simulink model "CTS_inequality_2021b"  (R2021b)
settings: Solver=FixedStepAuto  StartTime=0.0  StopTime=300  FixedStep=0.01  RelTol=1e-3
settings Model: PacingRate=0.200000  Creator=25307  LastModifiedBy=25307
settings DebuggingCC: UnconnectedInputMsg=none  UnconnectedOutputMsg=none  UnconnectedLineMsg=none
settings ModelReferenceCC: EnableRefExpFcnMdlSchedulingChecks=off
settings RTWCC: DLArmComputeVersion=20.02.1

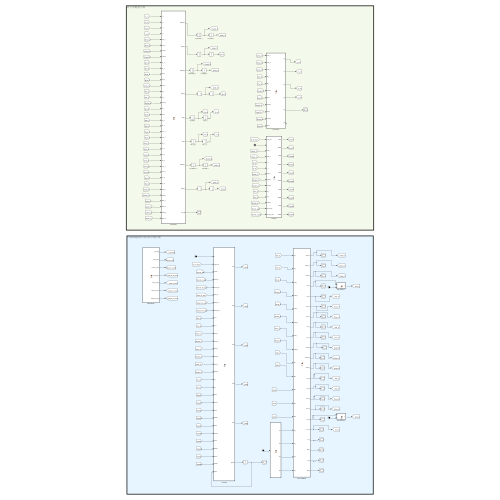
[thumbnail: Simulink's stored preview of the top-level diagram]
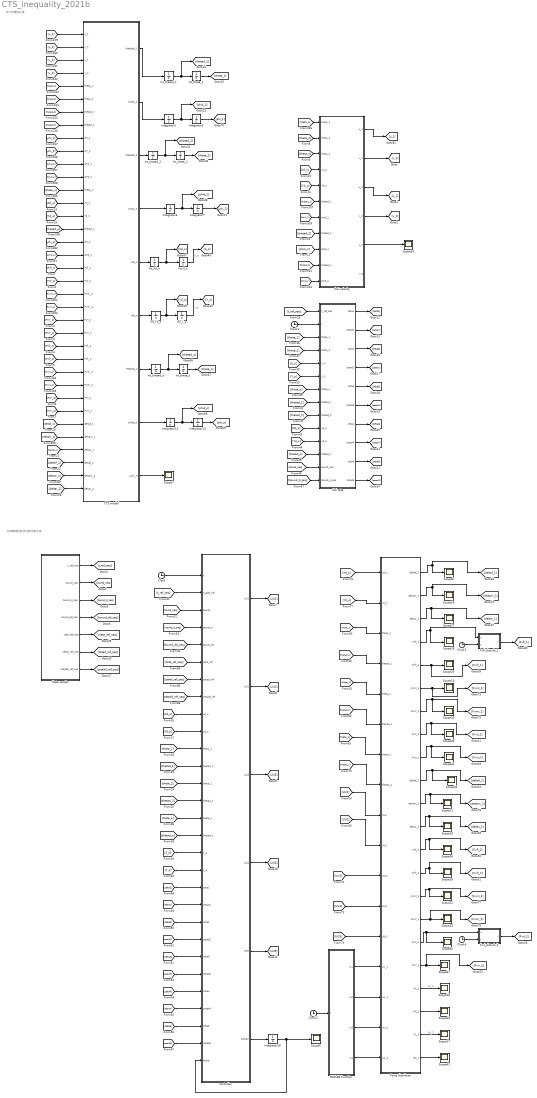
== system CTS_inequality_2021b ==
  note: 动力学模型区域
  note: 约束跟随控制及控制分配区域
  CTS model : MATLAB Function  TreatAsAtomicUnit=on
  Cal velocity : MATLAB Function  TreatAsAtomicUnit=on
  Cal zeta : MATLAB Function  TreatAsAtomicUnit=on
  Clock{,1..4} (5 alike) : Clock
  Data sender : MATLAB Function  TreatAsAtomicUnit=on
  Force distribute : MATLAB Function  TreatAsAtomicUnit=on
  Fxfl_disturb_1 : MATLAB Function  TreatAsAtomicUnit=on
  Fxrl_disturb_2 : MATLAB Function  TreatAsAtomicUnit=on
  Int_X_o : Integrator  InitialCondition=32.7448
  Int_Xd_o : Integrator  InitialCondition=1.1
  Int_Y_o : Integrator  InitialCondition=12.2889
  Int_Yd_o : Integrator  InitialCondition=0.0024
  Int_theta_1 : Integrator
  Int_theta_2 : Integrator  InitialCondition=0.005
  Int_theta_o : Integrator  InitialCondition=0.0014
  Int_thetad_1 : Integrator
  Int_thetad_2 : Integrator  InitialCondition=-0.0031
  Int_thetad_o : Integrator  InitialCondition=-0.001
  Integrator{2..3,6..7,12..13} (6 alike) : Integrator
  Integrator16 : Integrator  InitialCondition=0.5
  MATLAB Function : MATLAB Function  TreatAsAtomicUnit=on
  Scope{5..7,16..24,27..37,40..41} (25 alike) : Scope
  controller : MATLAB Function  TreatAsAtomicUnit=on
  wires:
  [theta_o] -> Cal velocity/3(theta_o)
  [thetad_1] -> CTS model/7(thetad_1)
  [theta_o] -> CTS model/13(theta_o)
  [theta_2] -> CTS model/6(theta_2)
  [phid_1] -> Cal velocity/7(phid_1)
  [Fxrl_1] -> CTS model/23(Fxrl_1)
  Integrator6/1 -> [phid_2], Integrator7/1
  [Fxfr_2] -> CTS model/26(Fxfr_2)
  [phi_o] -> CTS model/17(phi_o)
  [deltaf_2] -> CTS model/34(deltaf_2)
  [Yd_o] -> Cal velocity/5(Yd_o)
  [phi_2] -> CTS model/10(phi_2)
  [theta_1] -> Cal velocity/1(theta_1)
  [Fxrl_2] -> CTS model/29(Fxrl_2)
  [theta_2] -> Cal velocity/2(theta_2)
  [phid_1] -> CTS model/11(phid_1)
  Integrator3/1 -> [phi_1]
  [v_1] -> CTS model/3(v_1)
  CTS model/8(phidd_o) -> Integrator12/1
  [Xd_o] -> Cal velocity/4(Xd_o)
  [thetad_2] -> CTS model/8(thetad_2)
  [phid_2] -> Cal velocity/9(phid_2)
  [phid_2] -> CTS model/12(phid_2)
  [Xd_o] -> CTS model/14(Xd_o)
  Cal velocity/2(v_1) -> [v_1]
  [thetad_1] -> Cal velocity/6(thetad_1)
  [deltar_1] -> CTS model/33(deltar_1)
  Cal velocity/4(v_2) -> [v_2]
  [u_1] -> CTS model/1(u_1)
  Integrator12/1 -> [phid_o], Integrator13/1
  [Fxfl_1] -> CTS model/19(Fxfl_1)
  [Fxrr_2] -> CTS model/30(Fxrr_2)
  [deltaf_1] -> CTS model/31(deltaf_1)
  [thetad_o] -> Cal velocity/10(thetad_o)
  [Fxrr_1] -> CTS model/24(Fxrr_1)
  Cal velocity/1(u_1) -> [u_1]
  Integrator13/1 -> [phi_o]
  [phid_o] -> CTS model/18(phid_o)
  CTS model/4(phidd_2) -> Integrator6/1
  CTS model/9(rank_M) -> Scope7/1
  Integrator7/1 -> [phi_2]
  [u_2] -> CTS model/2(u_2)
  [Fxfl_2] -> CTS model/25(Fxfl_2)
  [thetad_2] -> Cal velocity/8(thetad_2)
  [v_2] -> CTS model/4(v_2)
  [Yd_o] -> CTS model/15(Yd_o)
  [phi_1] -> CTS model/9(phi_1)
  [theta_1] -> CTS model/5(theta_1)
  [thetad_o] -> CTS model/16(thetad_o)
  Integrator2/1 -> [phid_1], Integrator3/1
  [deltar_2] -> CTS model/36(deltar_2)
  CTS model/2(phidd_1) -> Integrator2/1
  [Fxfr_1] -> CTS model/20(Fxfr_1)
  [phid_o] -> Cal velocity/11(phid_o)
  Cal velocity/3(u_2) -> [u_2]
  [bound_d_seq] -> controller/4(bound_d)
  [zetadd_ref_seq] -> controller/8(zetadd_ref)
  [bound_dd_seq] -> controller/5(bound_dd)
  controller/6(alphad) -> Integrator16/1
  Data sender/5(zeta_ref_seq) -> [zeta_ref_seq]
  [zetad2] -> controller/22(zetad2)
  Data sender/7(zetadd_ref_seq) -> [zetadd_ref_seq]
  [theta_o] -> Force distribute/7(theta_o)
  Data sender/6(zetad_ref_seq) -> [zetad_ref_seq]
  [theta_1] -> Force distribute/3(theta_1)
  [zeta_ref_seq] -> controller/6(zeta_ref)
  [zetad_ref_seq] -> controller/7(zetad_ref)
  Force distribute/4(Fxfl_1) -> Scope28/1, Fxfl_disturb_1/1(u)
  Data sender/3(bound_d_seq) -> [bound_d_seq]
  [zetad4] -> controller/26(zetad4)
  [zetad3] -> controller/24(zetad3)
  controller/4(UU4) -> [UU4]
  Clock/1 -> controller/1(t)
  [zetad5] -> controller/28(zetad5)
  [bound_seq] -> controller/3(bound)
  [thetad_o] -> Force distribute/8(thetad_o)
  [zeta3] -> controller/23(zeta3)
  Integrator16/1 -> Scope5/1, controller/29(alpha)
  [zeta4] -> controller/25(zeta4)
  [UU5] -> Force distribute/13(UU5)
  controller/5(UU5) -> [UU5]
  [theta_o] -> controller/15(theta_o)
  [X_o] -> controller/17(x_o)
  [zeta1] -> controller/19(zeta1)
  controller/3(UU3) -> [UU3]
  Data sender/1(t_ref_seq) -> [t_ref_seq]
  [t_ref_seq] -> controller/2(t_glob_ref)
  Force distribute/1(deltaf_1) -> Scope6/1, [deltaf_1]
  [thetad_2] -> controller/14(thetad_2)
  [theta_1] -> controller/11(theta_1)
  [Xd_o] -> controller/9(xd_o)
  Force distribute/12(deltar_2) -> Scope33/1, [deltar_2]
  [Y_o] -> controller/18(y_o)
  [thetad_1] -> controller/12(thetad_1)
  [Yd_o] -> controller/10(yd_o)
  Data sender/2(bound_seq) -> [bound_seq]
  [thetad_1] -> Force distribute/4(thetad_1)
  controller/1(UU1) -> [UU1]
  Force distribute/5(Fxfr_1) -> [Fxfr_1], Scope29/1
  Force distribute/18(Fxrr_2) -> [Fxrr_2], Scope37/1
  [theta_2] -> controller/13(theta_2)
  [UU4] -> Force distribute/12(UU4)
  [UU3] -> Force distribute/11(UU3)
  Force distribute/9(Fxrr_1) -> Scope31/1, [Fxrr_1]
  [zeta5] -> controller/27(zeta5)
  Force distribute/10(deltaf_2) -> Scope32/1, [deltaf_2]
  [UU1] -> Force distribute/9(UU1)
  [zetad1] -> controller/20(zetad1)
  [zeta2] -> controller/21(zeta2)
  [thetad_2] -> Force distribute/6(thetad_2)
  [Yd_o] -> Force distribute/2(yd_o)
  [thetad_o] -> controller/16(thetad_o)
  Force distribute/8(Fxrl_1) -> Scope30/1, [Fxrl_1]
  Data sender/4(bound_dd_seq) -> [bound_dd_seq]
  Force distribute/14(Fxfr_2) -> Scope35/1, [Fxfr_2]
  controller/2(UU2) -> [UU2]
  Force distribute/13(Fxfl_2) -> Scope34/1, [Fxfl_2]
  [theta_2] -> Force distribute/5(theta_2)
  [Xd_o] -> Force distribute/1(xd_o)
  [UU2] -> Force distribute/10(UU2)
  Cal zeta/3(zeta2) -> [zeta2]
  Cal zeta/10(zetad5) -> [zetad5]
  [t_ref_seq] -> Cal zeta/1(t_ref_seq)
  Cal zeta/8(zetad4) -> [zetad4]
  [Xd_o] -> Cal zeta/10(xd_o)
  [theta_2] -> Cal zeta/4(theta_2)
  [theta_o] -> Cal zeta/7(theta_o)
  Cal zeta/7(zeta4) -> [zeta4]
  Cal zeta/2(zetad1) -> [zetad1]
  [Yd_o] -> Cal zeta/11(yd_o)
  [X_o] -> Cal zeta/5(x_o)
  Cal zeta/1(zeta1) -> [zeta1]
  [thetad_2] -> Cal zeta/9(thetad_2)
  [bound_d_seq] -> Cal zeta/14(bound_d_seq)
  [thetad_1] -> Cal zeta/8(thetad_1)
  Cal zeta/9(zeta5) -> [zeta5]
  [Y_o] -> Cal zeta/6(y_o)
  [bound_seq] -> Cal zeta/13(bound_seq)
  Cal zeta/5(zeta3) -> [zeta3]
  Cal zeta/4(zetad2) -> [zetad2]
  [thetad_o] -> Cal zeta/12(thetad_o)
  [theta_1] -> Cal zeta/3(theta_1)
  Clock1/1 -> Cal zeta/2(t)
  Cal zeta/6(zetad3) -> [zetad3]
  Int_theta_1/1 -> [theta_1]
  CTS model/1(thetadd_1) -> Int_thetad_1/1
  Int_thetad_1/1 -> [thetad_1], Int_theta_1/1
  Int_thetad_2/1 -> [thetad_2], Int_theta_2/1
  Int_theta_2/1 -> [theta_2]
  CTS model/3(thetadd_2) -> Int_thetad_2/1
  CTS model/5(Xdd_o) -> Int_Xd_o/1
  Int_Xd_o/1 -> Int_X_o/1, [Xd_o]
  Int_X_o/1 -> [X_o]  "X_o"
  Int_Y_o/1 -> [Y_o]  "Y_o"
  Int_Yd_o/1 -> Int_Y_o/1, [Yd_o]
  CTS model/6(Ydd_o) -> Int_Yd_o/1
  CTS model/7(thetadd_o) -> Int_thetad_o/1
  Int_thetad_o/1 -> [thetad_o], Int_theta_o/1
  Int_theta_o/1 -> [theta_o]
  MATLAB Function/1(w1) -> Force distribute/14(wx_1)
  MATLAB Function/2(w2) -> Force distribute/15(wz_1)
  MATLAB Function/3(w3) -> Force distribute/16(wx_2)
  MATLAB Function/4(w4) -> Force distribute/17(wz_2)
  Clock2/1 -> MATLAB Function/1(t)
  Clock3/1 -> Fxfl_disturb_1/2(t)
  Fxfl_disturb_1/1(y) -> [Fxfl_1]
  Clock4/1 -> Fxrl_disturb_2/2(t)
  Fxrl_disturb_2/1(y) -> [Fxrl_2]
  Force distribute/17(Fxrl_2) -> Scope36/1, Fxrl_disturb_2/1(u)
  Force distribute/19(Fx_1) -> Scope16/1  "Fx_1"
  Force distribute/21(Fx_2) -> Scope17/1  "Fx_2"
  Force distribute/2(deltam_1) -> Scope18/1, [deltam_1]
  Force distribute/7(Fxmr_1) -> Scope20/1, [Fxmr_1]
  Force distribute/6(Fxml_1) -> Scope19/1, [Fxml_1]
  Force distribute/11(deltam_2) -> Scope21/1, [deltam_2]
  Force distribute/15(Fxml_2) -> Scope22/1, [Fxml_2]
  Force distribute/16(Fxmr_2) -> [Fxmr_2], Scope23/1
  [Fxml_1] -> CTS model/21(Fxml_1)
  [Fxmr_1] -> CTS model/22(Fxmr_1)
  [Fxml_2] -> CTS model/27(Fxml_2)
  [Fxmr_2] -> CTS model/28(Fxmr_2)
  [deltam_1] -> CTS model/32(deltam_1)
  [deltam_2] -> CTS model/35(deltam_2)
  Cal velocity/5(u_o) -> Scope24/1
  Force distribute/3(deltar_1) -> Scope27/1, [deltar_1]
  Force distribute/20(MZ_1) -> Scope40/1
  Force distribute/22(MZ_2) -> Scope41/1

== matlab function CTS_inequality_2021b/Cal zeta ==
  data: t_ref_seq input; zeta1 output; t input; theta_1 input; theta_2 input; x_o input; y_o input; theta_o input; thetad_1 input; thetad_2 input; xd_o input; yd_o input; thetad_o input; bound_seq input; bound_d_seq input; zetad1 output; zeta2 output; zetad2 output; zeta3 output; zetad3 output; zeta4 output; zetad4 output; zeta5 output; zetad5 output
function [zeta1,zetad1,zeta2,zetad2,zeta3,zetad3,zeta4,zetad4,zeta5,zetad5] = fcn(t_ref_seq,t,theta_1,theta_2,x_o,y_o,theta_o,thetad_1,thetad_2,xd_o,yd_o,thetad_o,bound_seq,bound_d_seq)

x_hi_all_o = bound_seq(1,:);
x_lo_all_o = bound_seq(2,:);
y_hi_all_o = bound_seq(3,:);
y_lo_all_o = bound_seq(4,:);
theta_hi_all_o = bound_seq(5,:);
theta_lo_all_o = bound_seq(6,:);
theta_hi_all_1 = bound_seq(7,:);
theta_lo_all_1 = bound_seq(8,:);
theta_hi_all_2 = bound_seq(9,:);
theta_lo_all_2 = bound_seq(10,:);

xd_hi_all_o = bound_d_seq(1,:);
xd_lo_all_o = bound_d_seq(2,:);
yd_hi_all_o = bound_d_seq(3,:);
yd_lo_all_o = bound_d_seq(4,:);
thetad_hi_all_o = bound_d_seq(5,:);
thetad_lo_all_o = bound_d_seq(6,:);
thetad_hi_all_1 = bound_d_seq(7,:);
thetad_lo_all_1 = bound_d_seq(8,:);
thetad_hi_all_2 = bound_d_seq(9,:);
thetad_lo_all_2 = bound_d_seq(10,:);


x_hi_o = spline(t_ref_seq,x_hi_all_o,t);
x_lo_o = spline(t_ref_seq,x_lo_all_o,t);
y_hi_o = spline(t_ref_seq,y_hi_all_o,t);
y_lo_o = spline(t_ref_seq,y_lo_all_o,t);
theta_hi_o = spline(t_ref_seq,theta_hi_all_o,t);
theta_lo_o = spline(t_ref_seq,theta_lo_all_o,t);
theta_hi_1 = spline(t_ref_seq,theta_hi_all_1,t);
theta_lo_1 = spline(t_ref_seq,theta_lo_all_1,t);
theta_hi_2 = spline(t_ref_seq,theta_hi_all_2,t);
theta_lo_2 = spline(t_ref_seq,theta_lo_all_2,t);

xd_hi_o = spline(t_ref_seq,xd_hi_all_o,t);
xd_lo_o = spline(t_ref_seq,xd_lo_all_o,t);
yd_hi_o = spline(t_ref_seq,yd_hi_all_o,t);
yd_lo_o = spline(t_ref_seq,yd_lo_all_o,t);
thetad_hi_o = spline(t_ref_seq,thetad_hi_all_o,t);
thetad_lo_o = spline(t_ref_seq,thetad_lo_all_o,t);
thetad_hi_1 = spline(t_ref_seq,thetad_hi_all_1,t);
thetad_lo_1 = spline(t_ref_seq,thetad_lo_all_1,t);
thetad_hi_2 = spline(t_ref_seq,thetad_hi_all_2,t);
thetad_lo_2 = spline(t_ref_seq,thetad_lo_all_2,t);

zeta1 = log((theta_1-theta_lo_1)/(theta_hi_1-theta_1));
zeta2 = log((theta_2-theta_lo_2)/(theta_hi_2-theta_2));
zeta3 = log((x_o-x_lo_o)/(x_hi_o-x_o));
zeta4 = log((y_o-y_lo_o)/(y_hi_o-y_o));
zeta5 = log((theta_o-theta_lo_o)/(theta_hi_o-theta_o));

zetad1 = (((thetad_1-thetad_lo_1)/(theta_1-theta_hi_1)-((thetad_1-thetad_hi_1)*(theta_1-theta_lo_1))/(theta_1-theta_hi_1)^2)*(theta_1-theta_hi_1))/(theta_1-theta_lo_1);
zetad2 = (((thetad_2-thetad_lo_2)/(theta_2-theta_hi_2)-((thetad_2-thetad_hi_2)*(theta_2-theta_lo_2))/(theta_2-theta_hi_2)^2)*(theta_2-theta_hi_2))/(theta_2-theta_lo_2);
zetad3 = (((xd_o-xd_lo_o)/(x_o-x_hi_o)-((xd_o-xd_hi_o)*(x_o-x_lo_o))/(x_o-x_hi_o)^2)*(x_o-x_hi_o))/(x_o-x_lo_o);
zetad4 = (((yd_o-yd_lo_o)/(y_o-y_hi_o)-((yd_o-yd_hi_o)*(y_o-y_lo_o))/(y_o-y_hi_o)^2)*(y_o-y_hi_o))/(y_o-y_lo_o);
zetad5 = (((thetad_o-thetad_lo_o)/(theta_o-theta_hi_o)-((thetad_o-thetad_hi_o)*(theta_o-theta_lo_o))/(theta_o-theta_hi_o)^2)*(theta_o-theta_hi_o))/(theta_o-theta_lo_o);

== matlab function CTS_inequality_2021b/CTS model ==
  data: thetadd_1 output; phidd_1 output; thetadd_2 output; phidd_2 output; Xdd_o output; Ydd_o output; thetadd_o output; phidd_o output; u_1 input; u_2 input; v_1 input; v_2 input; theta_1 input; theta_2 input; thetad_1 input; thetad_2 input; phi_1 input; phi_2 input; phid_1 input; phid_2 input; theta_o input; Xd_o input; Yd_o input; thetad_o input; phi_o input; phid_o input; Fxfl_1 input; Fxfr_1 input; Fxml_1 input; Fxmr_1 input; Fxrl_1 input; Fxrr_1 input; Fxfl_2 input; Fxfr_2 input; Fxml_2 input; Fxmr_2 input; Fxrl_2 input; Fxrr_2 input; rank_M output; deltaf_1 input; deltam_1 input; deltar_1 input; deltaf_2 input; deltam_2 input; deltar_2 input
function [thetadd_1,phidd_1,thetadd_2,phidd_2,Xdd_o,Ydd_o,thetadd_o,phidd_o,rank_M] = fcn(u_1,u_2,v_1,v_2,theta_1,theta_2,thetad_1,thetad_2,phi_1,phi_2,phid_1,phid_2,theta_o,Xd_o,Yd_o,thetad_o,phi_o,phid_o,...
    Fxfl_1,Fxfr_1,Fxml_1,Fxmr_1,Fxrl_1,Fxrr_1,Fxfl_2,Fxfr_2,Fxml_2,Fxmr_2,Fxrl_2,Fxrr_2,deltaf_1,deltam_1,deltar_1,deltaf_2,deltam_2,deltar_2)



m_1 = 4455;
Iz_1 = 26802.6;
a_1 = 1.11;
b_1 = 0.12;
c_1 = 1.23;
d_1 = 0.5;
r_1 = 5;
phip_1 = 0;
Cf_1 = -87752;
Cm_1 = -82100;
Cr_1 = -88752;
ms_1 = 4155;
Ix_1 = 2283.9;
K_1 = 253750;
C_1 = 15225;
hs_1 = 0.65;
hcr_1 = 1;


m_2 = 5925;
Iz_2 = 24802.6;
a_2 = 1.11;
b_2 = 0.12;
c_2 = 1.23;
d_2 = 0.5;
r_2 = 5;
phip_2 = pi;
Cf_2 = -86752;
Cm_2 = -83222;
Cr_2 = -85752;
ms_2 = 5455;
Ix_2 = 2283.9;
K_2 = 253750;
C_2 = 15225;
hs_2 = 0.65;
hcr_2 = 1;

m_o = 5925;
Iz_o = 65992;
Ix_o = 4690;
H_o = 1.5;
Kj = 333023;
Cj = 45023;
g = 9.81;

T_1 = 1.5;
T_2 = 1.5;

hr = 0.2;


Fx_1 = Fxfl_1+Fxfr_1+Fxml_1+Fxmr_1+Fxrl_1+Fxrr_1;
Fy_1 = (Fxfl_1+Fxfr_1)*deltaf_1+(Fxml_1+Fxmr_1)*deltam_1+(Fxrl_1+Fxrr_1)*deltar_1;
Mz_1 = (Fxfl_1+Fxfr_1)*a_1*deltaf_1-(Fxfl_1-Fxfr_1)*T_1/2-(Fxml_1+Fxmr_1)*b_1*deltam_1-(Fxml_1-Fxmr_1)*T_1/2-(Fxrl_1+Fxrr_1)*c_1*deltar_1-(Fxrl_1-Fxrr_1)*T_1/2;

Q1_1 = m_1*v_1*thetad_1;
Q2_1 = -m_1*u_1*thetad_1+2*Cf_1*(v_1+thetad_1*a_1)/u_1+2*Cm_1*(v_1-thetad_1*b_1)/u_1+2*Cr_1*(v_1-thetad_1*c_1)/u_1;
Q3_1 = 2*Cf_1*(v_1+thetad_1*a_1)/u_1*a_1-2*Cm_1*(v_1-thetad_1*b_1)/u_1*b_1-2*Cr_1*(v_1-thetad_1*c_1)/u_1*c_1;
Q4_1 = -K_1*phi_1-C_1*phid_1+ms_1*g*(hs_1-hr)*phi_1+ms_1*(hs_1-hr)*u_1*thetad_1+Kj*(phi_o-phi_1)+Cj*(phid_o-phid_1);

U1_1 = -2*Cf_1*(v_1+thetad_1*a_1)/u_1*deltaf_1-2*Cm_1*(v_1-thetad_1*b_1)/u_1*deltam_1-2*Cr_1*(v_1-thetad_1*c_1)/u_1*deltar_1+Fx_1+2*(Cf_1*deltaf_1^2+Cm_1*deltam_1^2+Cr_1*deltar_1^2);
U2_1 = -2*Cf_1*deltaf_1-2*Cm_1*deltam_1-2*Cr_1*deltar_1+Fy_1;
U3_1 = -2*Cf_1*a_1*deltaf_1+2*Cm_1*b_1*deltam_1+2*Cr_1*c_1*deltar_1+Mz_1;


Fx_2 = Fxfl_2+Fxfr_2+Fxml_2+Fxmr_2+Fxrl_2+Fxrr_2;
Fy_2 = (Fxfl_2+Fxfr_2)*deltaf_2+(Fxml_2+Fxmr_2)*deltam_2+(Fxrl_2+Fxrr_2)*deltar_2;
Mz_2 = (Fxfl_2+Fxfr_2)*a_2*deltaf_2-(Fxfl_2-Fxfr_2)*T_2/2-(Fxml_2+Fxmr_2)*b_2*deltam_2-(Fxml_2-Fxmr_2)*T_2/2-(Fxrl_2+Fxrr_2)*c_2*deltar_2-(Fxrl_2-Fxrr_2)*T_2/2;

Q1_2 = m_2*v_2*thetad_2;
Q2_2 = -m_2*u_2*thetad_2+2*Cf_2*(v_2+thetad_2*a_2)/u_2+2*Cm_2*(v_2-thetad_2*b_2)/u_2+2*Cr_2*(v_2-thetad_2*c_2)/u_2;
Q3_2 = 2*Cf_2*(v_2+thetad_2*a_2)/u_2*a_2-2*Cm_2*(v_2-thetad_2*b_2)/u_2*b_2-2*Cr_2*(v_2-thetad_2*c_2)/u_2*c_2;
Q4_2 = -K_2*phi_2-C_2*phid_2+ms_2*g*(hs_2-hr)*phi_2+ms_2*(hs_2-hr)*u_2*thetad_2+Kj*(phi_o-phi_2)+Cj*(phid_o-phid_2);

U1_2 = -2*Cf_2*(v_2+thetad_2*a_2)/u_2*deltaf_2-2*Cm_2*(v_2-thetad_2*b_2)/u_2*deltam_2-2*Cr_2*(v_2-thetad_2*c_2)/u_2*deltar_2+Fx_2+2*(Cf_2*deltaf_2^2+Cm_2*deltam_2^2+Cr_2*deltar_2^2);
U2_2 = -2*Cf_2*deltaf_2-2*Cm_2*deltam_2-2*Cr_2*deltar_2+Fy_2;
U3_2 = -2*Cf_2*a_2*deltaf_2+2*Cm_2*b_2*deltam_2+2*Cr_2*c_2*deltar_2+Mz_2;

Q4_o = -Kj*(phi_o-phi_1)-Kj*(phi_o-phi_2)-Cj*(phid_o-phid_1)-Cj*(phid_o-phid_2)+m_o*g*(H_o-hr)*phi_o;


M = zeros(8,8);
M(1,1) = (m_1*d_1^2+Iz_1);
M(1,2) = +(d_1*hr*m_1-d_1*hcr_1*m_1-d_1*hr*ms_1+d_1*hs_1*ms_1);
M(1,3) = 0;
M(1,4) = 0;
M(1,5) = +(d_1*m_1*sin(theta_1));
M(1,6) = +(-d_1*m_1*cos(theta_1));
M(1,7) = +(-d_1*m_1*r_1*cos(phip_1-theta_1+theta_o));
M(1,8) = +(d_1*hcr_1*m_1*cos(theta_1-theta_o)-d_1*hr*m_1*cos(theta_1-theta_o));

M(2,1) = (d_1*hr*m_1-d_1*hcr_1*m_1-d_1*hr*ms_1+d_1*hs_1*ms_1);
M(2,2) = +(Ix_1+hcr_1^2*m_1+hr^2*m_1-hr^2*ms_1+hs_1^2*ms_1-2*hcr_1*hr*m_1+2*hcr_1*hr*ms_1-2*hcr_1*hs_1*ms_1);
M(2,3) = 0;
M(2,4) = 0;
M(2,5) = +(hr*m_1*sin(theta_1)-hcr_1*m_1*sin(theta_1)-hr*ms_1*sin(theta_1)+hs_1*ms_1*sin(theta_1));
M(2,6) = +(hcr_1*m_1*cos(theta_1)-hr*m_1*cos(theta_1)+hr*ms_1*cos(theta_1)-hs_1*ms_1*cos(theta_1));
M(2,7) = +(hcr_1*m_1*r_1*cos(phip_1-theta_1+theta_o)-hr*m_1*r_1*cos(phip_1-theta_1+theta_o)+hr*ms_1*r_1*cos(phip_1-theta_1+theta_o)-hs_1*ms_1*r_1*cos(phip_1-theta_1+theta_o));
M(2,8) = +(hr^2*ms_1*cos(theta_1-theta_o)-hr^2*m_1*cos(theta_1-theta_o)-hcr_1^2*m_1*cos(theta_1-theta_o)+2*hcr_1*hr*m_1*cos(theta_1-theta_o)-hcr_1*hr*ms_1*cos(theta_1-theta_o)+hcr_1*hs_1*ms_1*cos(theta_1-theta_o)-hr*hs_1*ms_1*cos(theta_1-theta_o));

M(3,1) = 0;
M(3,2) = 0;
M(3,3) = (m_2*d_2^2+Iz_2);
M(3,4) = +(d_2*hr*m_2-d_2*hcr_2*m_2-d_2*hr*ms_2+d_2*hs_2*ms_2);
M(3,5) = +(d_2*m_2*sin(theta_2));
M(3,6) = +(-d_2*m_2*cos(theta_2));
M(3,7) = +(-d_2*m_2*r_2*cos(phip_2-theta_2+theta_o));
M(3,8) = +(d_2*hcr_2*m_2*cos(theta_2-theta_o)-d_2*hr*m_2*cos(theta_2-theta_o));

M(4,1) = 0;
M(4,2) = 0;
M(4,3) = (d_2*hr*m_2-d_2*hcr_2*m_2-d_2*hr*ms_2+d_2*hs_2*ms_2);
M(4,4) = +(Ix_2+hcr_2^2*m_2+hr^2*m_2-hr^2*ms_2+hs_2^2*ms_2-2*hcr_2*hr*m_2+2*hcr_2*hr*ms_2-2*hcr_2*hs_2*ms_2);
M(4,5) = +(hr*m_2*sin(theta_2)-hcr_2*m_2*sin(theta_2)-hr*ms_2*sin(theta_2)+hs_2*ms_2*sin(theta_2));
M(4,6) = +(hcr_2*m_2*cos(theta_2)-hr*m_2*cos(theta_2)+hr*ms_2*cos(theta_2)-hs_2*ms_2*cos(theta_2));
M(4,7) = +(hcr_2*m_2*r_2*cos(phip_2-theta_2+theta_o)-hr*m_2*r_2*cos(phip_2-theta_2+theta_o)+hr*ms_2*r_2*cos(phip_2-theta_2+theta_o)-hs_2*ms_2*r_2*cos(phip_2-theta_2+theta_o));
M(4,8) = +(hr^2*ms_2*cos(theta_2-theta_o)-hr^2*m_2*cos(theta_2-theta_o)-hcr_2^2*m_2*cos(theta_2-theta_o)+2*hcr_2*hr*m_2*cos(theta_2-theta_o)-hcr_2*hr*ms_2*cos(theta_2-theta_o)+hcr_2*hs_2*ms_2*cos(theta_2-theta_o)-hr*hs_2*ms_2*cos(theta_2-theta_o));

M(5,1) = (d_1*m_1*sin(theta_1));
M(5,2) = +(hr*m_1*sin(theta_1)-hcr_1*m_1*sin(theta_1)-hr*ms_1*sin(theta_1)+hs_1*ms_1*sin(theta_1));
M(5,3) = +(d_2*m_2*sin(theta_2));
M(5,4) = +(hr*m_2*sin(theta_2)-hcr_2*m_2*sin(theta_2)-hr*ms_2*sin(theta_2)+hs_2*ms_2*sin(theta_2));
M(5,5) = +(m_1+m_2+m_o);
M(5,6) = 0;
M(5,7) = +(-m_1*r_1*sin(phip_1+theta_o)-m_2*r_2*sin(phip_2+theta_o));
M(5,8) = +(hcr_1*m_1*sin(theta_o)+hcr_2*m_2*sin(theta_o)-hr*m_1*sin(theta_o)-hr*m_2*sin(theta_o)-hr*m_o*sin(theta_o)+H_o*m_o*sin(theta_o));

M(6,1) = (-d_1*m_1*cos(theta_1));
M(6,2) = +(hcr_1*m_1*cos(theta_1)-hr*m_1*cos(theta_1)+hr*ms_1*cos(theta_1)-hs_1*ms_1*cos(theta_1));
M(6,3) = +(-d_2*m_2*cos(theta_2));
M(6,4) = +(hcr_2*m_2*cos(theta_2)-hr*m_2*cos(theta_2)+hr*ms_2*cos(theta_2)-hs_2*ms_2*cos(theta_2));
M(6,5) = 0;
M(6,6) = +(m_1+m_2+m_o);
M(6,7) = +(m_1*r_1*cos(phip_1+theta_o)+m_2*r_2*cos(phip_2+theta_o));
M(6,8) = +(hr*m_1*cos(theta_o)-hcr_2*m_2*cos(theta_o)-hcr_1*m_1*cos(theta_o)+hr*m_2*cos(theta_o)+hr*m_o*cos(theta_o)-H_o*m_o*cos(theta_o));

M(7,1) = (-d_1*m_1*r_1*cos(phip_1-theta_1+theta_o));
M(7,2) = +(hcr_1*m_1*r_1*cos(phip_1-theta_1+theta_o)-hr*m_1*r_1*cos(phip_1-theta_1+theta_o)+hr*ms_1*r_1*cos(phip_1-theta_1+theta_o)-hs_1*ms_1*r_1*cos(phip_1-theta_1+theta_o));
M(7,3) = +(-d_2*m_2*r_2*cos(phip_2-theta_2+theta_o));
M(7,4) = +(hcr_2*m_2*r_2*cos(phip_2-theta_2+theta_o)-hr*m_2*r_2*cos(phip_2-theta_2+theta_o)+hr*ms_2*r_2*cos(phip_2-theta_2+theta_o)-hs_2*ms_2*r_2*cos(phip_2-theta_2+theta_o));
M(7,5) = +(-m_1*r_1*sin(phip_1+theta_o)-m_2*r_2*sin(phip_2+theta_o));
M(7,6) = +(m_1*r_1*cos(phip_1+theta_o)+m_2*r_2*cos(phip_2+theta_o));
M(7,7) = +(m_1*r_1^2+m_2*r_2^2+Iz_o);
M(7,8) = +(hr*m_1*r_1*cos(phip_1)-hcr_2*m_2*r_2*cos(phip_2)-hcr_1*m_1*r_1*cos(phip_1)+hr*m_2*r_2*cos(phip_2));

M(8,1) = (d_1*hcr_1*m_1*cos(theta_1-theta_o)-d_1*hr*m_1*cos(theta_1-theta_o));
M(8,2) = +(hr^2*ms_1*cos(theta_1-theta_o)-hr^2*m_1*cos(theta_1-theta_o)-hcr_1^2*m_1*cos(theta_1-theta_o)+2*hcr_1*hr*m_1*cos(theta_1-theta_o)-hcr_1*hr*ms_1*cos(theta_1-theta_o)+hcr_1*hs_1*ms_1*cos(theta_1-theta_o)-hr*hs_1*ms_1*cos(theta_1-theta_o));
M(8,3) = +(d_2*hcr_2*m_2*cos(theta_2-theta_o)-d_2*hr*m_2*cos(theta_2-theta_o));
M(8,4) = +(hr^2*ms_2*cos(theta_2-theta_o)-hr^2*m_2*cos(theta_2-theta_o)-hcr_2^2*m_2*cos(theta_2-theta_o)+2*hcr_2*hr*m_2*cos(theta_2-theta_o)-hcr_2*hr*ms_2*cos(theta_2-theta_o)+hcr_2*hs_2*ms_2*cos(theta_2-theta_o)-hr*hs_2*ms_2*cos(theta_2-theta_o));
M(8,5) = +(hcr_1*m_1*sin(theta_o)+hcr_2*m_2*sin(theta_o)-hr*m_1*sin(theta_o)-hr*m_2*sin(theta_o)-hr*m_o*sin(theta_o)+H_o*m_o*sin(theta_o));
M(8,6) = +(hr*m_1*cos(theta_o)-hcr_2*m_2*cos(theta_o)-hcr_1*m_1*cos(theta_o)+hr*m_2*cos(theta_o)+hr*m_o*cos(theta_o)-H_o*m_o*cos(theta_o));
M(8,7) = +(hr*m_1*r_1*cos(phip_1)-hcr_2*m_2*r_2*cos(phip_2)-hcr_1*m_1*r_1*cos(phip_1)+hr*m_2*r_2*cos(phip_2));
M(8,8) = +(Ix_o+H_o^2*m_o+hcr_1^2*m_1+hcr_2^2*m_2+hr^2*m_1+hr^2*m_2+hr^2*m_o-2*H_o*hr*m_o-2*hcr_1*hr*m_1-2*hcr_2*hr*m_2);


Q_U = zeros(8,1);
Q_U(1) = -(+Q2_1*d_1-U3_1-Q3_1+U2_1*d_1+d_1*m_1*thetad_1*u_1-d_1*m_1*thetad_o*u_1+Xd_o*d_1*m_1*thetad_o*cos(theta_1)+Yd_o*d_1*m_1*thetad_o*sin(theta_1));
Q_U(2) = -(+Q2_1*hr-Q2_1*hcr_1-Q4_1-U2_1*hcr_1+U2_1*hr-hcr_1*m_1*thetad_1*u_1+hcr_1*m_1*thetad_o*u_1+hr*m_1*thetad_1*u_1-hr*m_1*thetad_o*u_1-hr*ms_1*thetad_1*u_1+hr*ms_1*thetad_o*u_1+hs_1*ms_1*thetad_1*u_1-hs_1*ms_1*thetad_o*u_1-Xd_o*hcr_1*m_1*thetad_o*cos(theta_1)+Xd_o*hr*m_1*thetad_o*cos(theta_1)-Xd_o*hr*ms_1*thetad_o*cos(theta_1)+Xd_o*hs_1*ms_1*thetad_o*cos(theta_1)-Yd_o*hcr_1*m_1*thetad_o*sin(theta_1)+Yd_o*hr*m_1*thetad_o*sin(theta_1)-Yd_o*hr*ms_1*thetad_o*sin(theta_1)+Yd_o*hs_1*ms_1*thetad_o*sin(theta_1));
Q_U(3) = -(+Q2_2*d_2-U3_2-Q3_2+U2_2*d_2+d_2*m_2*thetad_2*u_2-d_2*m_2*thetad_o*u_2+Xd_o*d_2*m_2*thetad_o*cos(theta_2)+Yd_o*d_2*m_2*thetad_o*sin(theta_2));
Q_U(4) = -(+Q2_2*hr-Q2_2*hcr_2-Q4_2-U2_2*hcr_2+U2_2*hr-hcr_2*m_2*thetad_2*u_2+hcr_2*m_2*thetad_o*u_2+hr*m_2*thetad_2*u_2-hr*m_2*thetad_o*u_2-hr*ms_2*thetad_2*u_2+hr*ms_2*thetad_o*u_2+hs_2*ms_2*thetad_2*u_2-hs_2*ms_2*thetad_o*u_2-Xd_o*hcr_2*m_2*thetad_o*cos(theta_2)+Xd_o*hr*m_2*thetad_o*cos(theta_2)-Xd_o*hr*ms_2*thetad_o*cos(theta_2)+Xd_o*hs_2*ms_2*thetad_o*cos(theta_2)-Yd_o*hcr_2*m_2*thetad_o*sin(theta_2)+Yd_o*hr*m_2*thetad_o*sin(theta_2)-Yd_o*hr*ms_2*thetad_o*sin(theta_2)+Yd_o*hs_2*ms_2*thetad_o*sin(theta_2));
Q_U(5) = -(+Q2_1*sin(theta_1)-Q1_2*cos(theta_2)-U1_1*cos(theta_1)-U1_2*cos(theta_2)-Q1_1*cos(theta_1)+Q2_2*sin(theta_2)+U2_1*sin(theta_1)+U2_2*sin(theta_2)+Yd_o*m_1*thetad_o+Yd_o*m_2*thetad_o+m_1*thetad_1*v_1*cos(theta_1)+m_2*thetad_2*v_2*cos(theta_2)-m_1*thetad_o*v_1*cos(theta_1)-m_2*thetad_o*v_2*cos(theta_2)+m_1*thetad_1*u_1*sin(theta_1)+m_2*thetad_2*u_2*sin(theta_2)-m_1*thetad_o*u_1*sin(theta_1)-m_2*thetad_o*u_2*sin(theta_2)+d_1*m_1*thetad_1^2*cos(theta_1)+d_2*m_2*thetad_2^2*cos(theta_2)-d_1*m_1*thetad_1*thetad_o*cos(theta_1)-d_2*m_2*thetad_2*thetad_o*cos(theta_2)-hcr_1*m_1*phid_1*thetad_1*cos(theta_1)-hcr_2*m_2*phid_2*thetad_2*cos(theta_2)+hcr_1*m_1*phid_1*thetad_o*cos(theta_1)+hcr_2*m_2*phid_2*thetad_o*cos(theta_2)+hr*m_1*phid_1*thetad_1*cos(theta_1)+hr*m_2*phid_2*thetad_2*cos(theta_2)-hr*m_1*phid_1*thetad_o*cos(theta_1)-hr*m_2*phid_2*thetad_o*cos(theta_2));
Q_U(6) = -(+m_1*thetad_o*u_1*cos(theta_1)-Q2_2*cos(theta_2)-U2_1*cos(theta_1)-U2_2*cos(theta_2)-Q1_1*sin(theta_1)-Q1_2*sin(theta_2)-U1_1*sin(theta_1)-U1_2*sin(theta_2)-Xd_o*m_1*thetad_o-Xd_o*m_2*thetad_o-m_1*thetad_1*u_1*cos(theta_1)-m_2*thetad_2*u_2*cos(theta_2)-Q2_1*cos(theta_1)+m_2*thetad_o*u_2*cos(theta_2)+m_1*thetad_1*v_1*sin(theta_1)+m_2*thetad_2*v_2*sin(theta_2)-m_1*thetad_o*v_1*sin(theta_1)-m_2*thetad_o*v_2*sin(theta_2)+d_1*m_1*thetad_1^2*sin(theta_1)+d_2*m_2*thetad_2^2*sin(theta_2)-d_1*m_1*thetad_1*thetad_o*sin(theta_1)-d_2*m_2*thetad_2*thetad_o*sin(theta_2)-hcr_1*m_1*phid_1*thetad_1*sin(theta_1)-hcr_2*m_2*phid_2*thetad_2*sin(theta_2)+hcr_1*m_1*phid_1*thetad_o*sin(theta_1)+hcr_2*m_2*phid_2*thetad_o*sin(theta_2)+hr*m_1*phid_1*thetad_1*sin(theta_1)+hr*m_2*phid_2*thetad_2*sin(theta_2)-hr*m_1*phid_1*thetad_o*sin(theta_1)-hr*m_2*phid_2*thetad_o*sin(theta_2));
Q_U(7) = -(+Q1_1*r_1*sin(phip_1-theta_1+theta_o)-Q2_2*r_2*cos(phip_2-theta_2+theta_o)-U2_1*r_1*cos(phip_1-theta_1+theta_o)-U2_2*r_2*cos(phip_2-theta_2+theta_o)-Q2_1*r_1*cos(phip_1-theta_1+theta_o)+Q1_2*r_2*sin(phip_2-theta_2+theta_o)+U1_1*r_1*sin(phip_1-theta_1+theta_o)+U1_2*r_2*sin(phip_2-theta_2+theta_o)-d_1*m_1*r_1*thetad_1^2*sin(phip_1-theta_1+theta_o)-d_2*m_2*r_2*thetad_2^2*sin(phip_2-theta_2+theta_o)-m_1*r_1*thetad_1*u_1*cos(phip_1-theta_1+theta_o)-m_2*r_2*thetad_2*u_2*cos(phip_2-theta_2+theta_o)+m_1*r_1*thetad_o*u_1*cos(phip_1-theta_1+theta_o)+m_2*r_2*thetad_o*u_2*cos(phip_2-theta_2+theta_o)-Xd_o*m_1*r_1*thetad_o*cos(phip_1+theta_o)-Xd_o*m_2*r_2*thetad_o*cos(phip_2+theta_o)-m_1*r_1*thetad_1*v_1*sin(phip_1-theta_1+theta_o)-m_2*r_2*thetad_2*v_2*sin(phip_2-theta_2+theta_o)+m_1*r_1*thetad_o*v_1*sin(phip_1-theta_1+theta_o)+m_2*r_2*thetad_o*v_2*sin(phip_2-theta_2+theta_o)-Yd_o*m_1*r_1*thetad_o*sin(phip_1+theta_o)-Yd_o*m_2*r_2*thetad_o*sin(phip_2+theta_o)+d_1*m_1*r_1*thetad_1*thetad_o*sin(phip_1-theta_1+theta_o)+d_2*m_2*r_2*thetad_2*thetad_o*sin(phip_2-theta_2+theta_o)+hcr_1*m_1*phid_1*r_1*thetad_1*sin(phip_1-theta_1+theta_o)+hcr_2*m_2*phid_2*r_2*thetad_2*sin(phip_2-theta_2+theta_o)-hcr_1*m_1*phid_1*r_1*thetad_o*sin(phip_1-theta_1+theta_o)-hcr_2*m_2*phid_2*r_2*thetad_o*sin(phip_2-theta_2+theta_o)-hr*m_1*phid_1*r_1*thetad_1*sin(phip_1-theta_1+theta_o)-hr*m_2*phid_2*r_2*thetad_2*sin(phip_2-theta_2+theta_o)+hr*m_1*phid_1*r_1*thetad_o*sin(phip_1-theta_1+theta_o)+hr*m_2*phid_2*r_2*thetad_o*sin(phip_2-theta_2+theta_o));
Q_U(8) = -(+Q2_1*hcr_1*cos(theta_1-theta_o)-Q4_o+Q2_2*hcr_2*cos(theta_2-theta_o)-Q2_1*hr*cos(theta_1-theta_o)-Q2_2*hr*cos(theta_2-theta_o)+U2_1*hcr_1*cos(theta_1-theta_o)+U2_2*hcr_2*cos(theta_2-theta_o)-U2_1*hr*cos(theta_1-theta_o)-U2_2*hr*cos(theta_2-theta_o)+Q1_1*hcr_1*sin(theta_1-theta_o)+Q1_2*hcr_2*sin(theta_2-theta_o)-Q1_1*hr*sin(theta_1-theta_o)-Q1_2*hr*sin(theta_2-theta_o)+U1_1*hcr_1*sin(theta_1-theta_o)+U1_2*hcr_2*sin(theta_2-theta_o)-U1_1*hr*sin(theta_1-theta_o)-U1_2*hr*sin(theta_2-theta_o)+hcr_1*m_1*thetad_1*u_1*cos(theta_1-theta_o)+hcr_2*m_2*thetad_2*u_2*cos(theta_2-theta_o)-hcr_1*m_1*thetad_o*u_1*cos(theta_1-theta_o)-hcr_2*m_2*thetad_o*u_2*cos(theta_2-theta_o)-hr*m_1*thetad_1*u_1*cos(theta_1-theta_o)-hr*m_2*thetad_2*u_2*cos(theta_2-theta_o)+hr*m_1*thetad_o*u_1*cos(theta_1-theta_o)+hr*m_2*thetad_o*u_2*cos(theta_2-theta_o)-hcr_1*m_1*thetad_1*v_1*sin(theta_1-theta_o)-hcr_2*m_2*thetad_2*v_2*sin(theta_2-theta_o)+hcr_1*m_1*thetad_o*v_1*sin(theta_1-theta_o)+hcr_2*m_2*thetad_o*v_2*sin(theta_2-theta_o)+hr*m_1*thetad_1*v_1*sin(theta_1-theta_o)+hr*m_2*thetad_2*v_2*sin(theta_2-theta_o)-hr*m_1*thetad_o*v_1*sin(theta_1-theta_o)-hr*m_2*thetad_o*v_2*sin(theta_2-theta_o)-d_1*hcr_1*m_1*thetad_1^2*sin(theta_1-theta_o)-d_2*hcr_2*m_2*thetad_2^2*sin(theta_2-theta_o)+d_1*hr*m_1*thetad_1^2*sin(theta_1-theta_o)+d_2*hr*m_2*thetad_2^2*sin(theta_2-theta_o)+hcr_1^2*m_1*phid_1*thetad_1*sin(theta_1-theta_o)+hcr_2^2*m_2*phid_2*thetad_2*sin(theta_2-theta_o)-hcr_1^2*m_1*phid_1*thetad_o*sin(theta_1-theta_o)-hcr_2^2*m_2*phid_2*thetad_o*sin(theta_2-theta_o)+hr^2*m_1*phid_1*thetad_1*sin(theta_1-theta_o)+hr^2*m_2*phid_2*thetad_2*sin(theta_2-theta_o)-hr^2*m_1*phid_1*thetad_o*sin(theta_1-theta_o)-hr^2*m_2*phid_2*thetad_o*sin(theta_2-theta_o)+Xd_o*hcr_1*m_1*thetad_o*cos(theta_o)+Xd_o*hcr_2*m_2*thetad_o*cos(theta_o)-Xd_o*hr*m_1*thetad_o*cos(theta_o)-Xd_o*hr*m_2*thetad_o*cos(theta_o)+Yd_o*hcr_1*m_1*thetad_o*sin(theta_o)+Yd_o*hcr_2*m_2*thetad_o*sin(theta_o)-Yd_o*hr*m_1*thetad_o*sin(theta_o)-Yd_o*hr*m_2*thetad_o*sin(theta_o)+d_1*hcr_1*m_1*thetad_1*thetad_o*sin(theta_1-theta_o)+d_2*hcr_2*m_2*thetad_2*thetad_o*sin(theta_2-theta_o)-d_1*hr*m_1*thetad_1*thetad_o*sin(theta_1-theta_o)-d_2*hr*m_2*thetad_2*thetad_o*sin(theta_2-theta_o)-2*hcr_1*hr*m_1*phid_1*thetad_1*sin(theta_1-theta_o)-2*hcr_2*hr*m_2*phid_2*thetad_2*sin(theta_2-theta_o)+2*hcr_1*hr*m_1*phid_1*thetad_o*sin(theta_1-theta_o)+2*hcr_2*hr*m_2*phid_2*thetad_o*sin(theta_2-theta_o));

qdd = M\(Q_U);

% Q_U = M*qdd

thetadd_1 = qdd(1);
phidd_1 = qdd(2);
thetadd_2 = qdd(3);
phidd_2 = qdd(4);
Xdd_o = qdd(5);
Ydd_o = qdd(6);
thetadd_o = qdd(7);
phidd_o = qdd(8);
rank_M = rank(M);

== matlab function CTS_inequality_2021b/controller ==
  data: t input; t_glob_ref input; UU1 output; bound input; bound_d input; bound_dd input; zeta_ref input; zetad_ref input; zetadd_ref input; UU2 output; UU3 output; UU4 output; UU5 output; xd_o input; yd_o input; theta_1 input; thetad_1 input; theta_2 input; thetad_2 input; theta_o input; thetad_o input; x_o input; y_o input; zeta1 input; zetad1 input; zeta2 input; zetad2 input; zeta3 input; zetad3 input; zeta4 input; zetad4 input; zeta5 input; zetad5 input; alpha input; alphad output
function [UU1,UU2,UU3,UU4,UU5,alphad] = fcn(t,t_glob_ref,bound,bound_d,bound_dd,zeta_ref,zetad_ref,zetadd_ref,...
    xd_o,yd_o,theta_1,thetad_1,theta_2,thetad_2,theta_o,thetad_o,x_o,y_o,zeta1,zetad1,zeta2,zetad2,zeta3,zetad3,zeta4,zetad4,zeta5,zetad5,alpha)


m_1 = 4455;
Iz_1 = 26802.6;
a_1 = 1.11;
b_1 = 0.12;
c_1 = 1.23;
d_1 = 0.5;
r_1 = 5;
phip_1 = 0;
Cf_1 = -89752;
Cm_1 = -82100;
Cr_1 = -89752;

m_2 = 5925;
Iz_2 = 24802.6;
a_2 = 1.11;
b_2 = 0.12;
c_2 = 1.23;
d_2 = 0.5;
r_2 = 5;
phip_2 = pi;
Cf_2 = -86752;
Cm_2 = -83222;
Cr_2 = -86752;

m_o = 5925;
Iz_o = 65992;

gamma = 10;
kappa = 2;

k1 = 0.02;
k2 = 0.002;
epsilon = 1;

zeta_ref_this1 = spline(t_glob_ref,zeta_ref(1,:),t);
zetad_ref_this1 = spline(t_glob_ref,zetad_ref(1,:),t);
zetadd_ref_this1 = spline(t_glob_ref,zetadd_ref(1,:),t);

zeta_ref_this2 = spline(t_glob_ref,zeta_ref(2,:),t);
zetad_ref_this2 = spline(t_glob_ref,zetad_ref(2,:),t);
zetadd_ref_this2 = spline(t_glob_ref,zetadd_ref(2,:),t);

zeta_ref_this3 = spline(t_glob_ref,zeta_ref(3,:),t);
zetad_ref_this3 = spline(t_glob_ref,zetad_ref(3,:),t);
zetadd_ref_this3 = spline(t_glob_ref,zetadd_ref(3,:),t);

zeta_ref_this4 = spline(t_glob_ref,zeta_ref(4,:),t);
zetad_ref_this4 = spline(t_glob_ref,zetad_ref(4,:),t);
zetadd_ref_this4 = spline(t_glob_ref,zetadd_ref(4,:),t);

zeta_ref_this5 = spline(t_glob_ref,zeta_ref(5,:),t);
zetad_ref_this5 = spline(t_glob_ref,zetad_ref(5,:),t);
zetadd_ref_this5 = spline(t_glob_ref,zetadd_ref(5,:),t);

x_hi_all_o = bound(1,:);
x_lo_all_o = bound(2,:);
y_hi_all_o = bound(3,:);
y_lo_all_o = bound(4,:);
theta_hi_all_o = bound(5,:);
theta_lo_all_o = bound(6,:);
theta_hi_all_1 = bound(7,:);
theta_lo_all_1 = bound(8,:);
theta_hi_all_2 = bound(9,:);
theta_lo_all_2 = bound(10,:);

xd_hi_all_o = bound_d(1,:);
xd_lo_all_o = bound_d(2,:);
yd_hi_all_o = bound_d(3,:);
yd_lo_all_o = bound_d(4,:);
thetad_hi_all_o = bound_d(5,:);
thetad_lo_all_o = bound_d(6,:);
thetad_hi_all_1 = bound_d(7,:);
thetad_lo_all_1 = bound_d(8,:);
thetad_hi_all_2 = bound_d(9,:);
thetad_lo_all_2 = bound_d(10,:);

xdd_hi_all_o = bound_dd(1,:);
xdd_lo_all_o = bound_dd(2,:);
ydd_hi_all_o = bound_dd(3,:);
ydd_lo_all_o = bound_dd(4,:);
thetadd_hi_all_o = bound_dd(5,:);
thetadd_lo_all_o = bound_dd(6,:);
thetadd_hi_all_1 = bound_dd(7,:);
thetadd_lo_all_1 = bound_dd(8,:);
thetadd_hi_all_2 = bound_dd(9,:);
thetadd_lo_all_2 = bound_dd(10,:);


x_hi_o = spline(t_glob_ref,x_hi_all_o,t);
x_lo_o = spline(t_glob_ref,x_lo_all_o,t);
y_hi_o = spline(t_glob_ref,y_hi_all_o,t);
y_lo_o = spline(t_glob_ref,y_lo_all_o,t);
theta_hi_o = spline(t_glob_ref,theta_hi_all_o,t);
theta_lo_o = spline(t_glob_ref,theta_lo_all_o,t);
theta_hi_1 = spline(t_glob_ref,theta_hi_all_1,t);
theta_lo_1 = spline(t_glob_ref,theta_lo_all_1,t);
theta_hi_2 = spline(t_glob_ref,theta_hi_all_2,t);
theta_lo_2 = spline(t_glob_ref,theta_lo_all_2,t);

xd_hi_o = spline(t_glob_ref,xd_hi_all_o,t);
xd_lo_o = spline(t_glob_ref,xd_lo_all_o,t);
yd_hi_o = spline(t_glob_ref,yd_hi_all_o,t);
yd_lo_o = spline(t_glob_ref,yd_lo_all_o,t);
thetad_hi_o = spline(t_glob_ref,thetad_hi_all_o,t);
thetad_lo_o = spline(t_glob_ref,thetad_lo_all_o,t);
thetad_hi_1 = spline(t_glob_ref,thetad_hi_all_1,t);
thetad_lo_1 = spline(t_glob_ref,thetad_lo_all_1,t);
thetad_hi_2 = spline(t_glob_ref,thetad_hi_all_2,t);
thetad_lo_2 = spline(t_glob_ref,thetad_lo_all_2,t);

xdd_hi_o = spline(t_glob_ref,xdd_hi_all_o,t);
xdd_lo_o = spline(t_glob_ref,xdd_lo_all_o,t);
ydd_hi_o = spline(t_glob_ref,ydd_hi_all_o,t);
ydd_lo_o = spline(t_glob_ref,ydd_lo_all_o,t);
thetadd_hi_o = spline(t_glob_ref,thetadd_hi_all_o,t);
thetadd_lo_o = spline(t_glob_ref,thetadd_lo_all_o,t);
thetadd_hi_1 = spline(t_glob_ref,thetadd_hi_all_1,t);
thetadd_lo_1 = spline(t_glob_ref,thetadd_lo_all_1,t);
thetadd_hi_2 = spline(t_glob_ref,thetadd_hi_all_2,t);
thetadd_lo_2 = spline(t_glob_ref,thetadd_lo_all_2,t);

xd_1 = xd_o-r_1*thetad_o*sin(theta_o+phip_1)+d_1*thetad_1*sin(theta_1);
yd_1 = yd_o+r_1*thetad_o*cos(theta_o+phip_1)-d_1*thetad_1*cos(theta_1);
xd_2 = xd_o-r_2*thetad_o*sin(theta_o+phip_2)+d_2*thetad_2*sin(theta_2);
yd_2 = yd_o+r_2*thetad_o*cos(theta_o+phip_2)-d_2*thetad_2*cos(theta_2);

u_1 = xd_1*cos(theta_1)+yd_1*sin(theta_1);
v_1 = -xd_1*sin(theta_1)+yd_1*cos(theta_1);
u_2 = xd_2*cos(theta_2)+yd_2*sin(theta_2);
v_2 = -xd_2*sin(theta_2)+yd_2*cos(theta_2);


Q1_1 = -2*Cf_1*(v_1+a_1*thetad_1)/u_1*sin(theta_1)-2*Cm_1*(v_1-b_1*thetad_1)/u_1*sin(theta_1)-2*Cr_1*(v_1-c_1*thetad_1)/u_1*sin(theta_1);
Q2_1 = 2*Cf_1*(v_1+a_1*thetad_1)/u_1*cos(theta_1)+2*Cm_1*(v_1-b_1*thetad_1)/u_1*cos(theta_1)+2*Cr_1*(v_1-c_1*thetad_1)/u_1*cos(theta_1);
Q3_1 = 2*Cf_1*(v_1+a_1*thetad_1)/u_1*a_1-2*Cm_1*(v_1-b_1*thetad_1)/u_1*b_1-2*Cr_1*(v_1-c_1*thetad_1)/u_1*c_1;

Q1_2 = -2*Cf_2*(v_2+a_2*thetad_2)/u_2*sin(theta_2)-2*Cm_2*(v_2-b_2*thetad_2)/u_2*sin(theta_2)-2*Cr_2*(v_2-c_2*thetad_2)/u_2*sin(theta_2);
Q2_2 = 2*Cf_2*(v_2+a_2*thetad_2)/u_2*cos(theta_2)+2*Cm_2*(v_2-b_2*thetad_2)/u_2*cos(theta_2)+2*Cr_2*(v_2-c_2*thetad_2)/u_2*cos(theta_2);
Q3_2 = 2*Cf_2*(v_2+a_2*thetad_2)/u_2*a_2-2*Cm_2*(v_2-b_2*thetad_2)/u_2*b_2-2*Cr_2*(v_2-c_2*thetad_2)/u_2*c_2;

M = [Iz_1+d_1^2*m_1,0,d_1*m_1*sin(theta_1),-d_1*m_1*cos(theta_1),-d_1*m_1*r_1*cos(phip_1-theta_1+theta_o);
    0,Iz_2+d_2^2*m_2,d_2*m_2*sin(theta_2),-d_2*m_2*cos(theta_2),-d_2*m_2*r_2*cos(phip_2-theta_2+theta_o);
    d_1*m_1*sin(theta_1),d_2*m_2*sin(theta_2),m_o+m_1+m_2,0,-m_1*r_1*sin(phip_1+theta_o)-m_2*r_2*sin(phip_2+theta_o);
    -d_1*m_1*cos(theta_1),-d_2*m_2*cos(theta_2),0,m_o+m_1+m_2,m_1*r_1*cos(phip_1+theta_o)+m_2*r_2*cos(phip_2+theta_o);
    -d_1*m_1*r_1*cos(phip_1-theta_1+theta_o),-d_2*m_2*r_2*cos(phip_2-theta_2+theta_o),-m_1*r_1*sin(phip_1+theta_o)-m_2*r_2*sin(phip_2+theta_o),m_1*r_1*cos(phip_1+theta_o)+m_2*r_2*cos(phip_2+theta_o),Iz_o+m_2*r_2^2+m_1*r_1^2];

QQ1 = Q3_1-Q2_1*d_1*cos(theta_1)+Q1_1*d_1*sin(theta_1)-d_1*m_1*r_1*thetad_o^2*sin(phip_1-theta_1+theta_o);
QQ2 = Q3_2-Q2_2*d_2*cos(theta_2)+Q1_2*d_2*sin(theta_2)-d_2*m_2*r_2*thetad_o^2*sin(phip_2-theta_2+theta_o);
QQ3 = Q1_1+Q1_2+m_1*r_1*thetad_o^2*cos(phip_1+theta_o)+m_2*r_2*thetad_o^2*cos(phip_2+theta_o)-d_1*m_1*thetad_1^2*cos(theta_1)-d_2*m_2*thetad_2^2*cos(theta_2);
QQ4 = Q2_1+Q2_2+m_1*r_1*thetad_o^2*sin(phip_1+theta_o)+m_2*r_2*thetad_o^2*sin(phip_2+theta_o)-d_1*m_1*thetad_1^2*sin(theta_1)-d_2*m_2*thetad_2^2*sin(theta_2);
QQ5 = Q2_1*r_1*cos(phip_1+theta_o)+Q2_2*r_2*cos(phip_2+theta_o)-Q1_1*r_1*sin(phip_1+theta_o)-Q1_2*r_2*sin(phip_2+theta_o)+d_1*m_1*r_1*thetad_1^2*sin(phip_1-theta_1+theta_o)+d_2*m_2*r_2*thetad_2^2*sin(phip_2-theta_2+theta_o);
QQ = [QQ1;QQ2;QQ3;QQ4;QQ5];

diff_phi_theta_1_theta_1 = -(((theta_1-theta_lo_1)/(theta_1-theta_hi_1)^2-1/(theta_1-theta_hi_1))*(theta_1-theta_hi_1))/(theta_1-theta_lo_1);
diff_phi_theta_1_theta_2 = 0;
diff_phi_theta_1_x_o = 0;
diff_phi_theta_1_y_o = 0;
diff_phi_theta_1_theta_o = 0;

diff_phi_theta_2_theta_1 = 0;
diff_phi_theta_2_theta_2 = -(((theta_2-theta_lo_2)/(theta_2-theta_hi_2)^2-1/(theta_2-theta_hi_2))*(theta_2-theta_hi_2))/(theta_2-theta_lo_2);
diff_phi_theta_2_x_o = 0;
diff_phi_theta_2_y_o = 0;
diff_phi_theta_2_theta_o = 0;

diff_phi_x_o_theta_1 = 0;
diff_phi_x_o_theta_2 = 0;
diff_phi_x_o_x_o = -(((x_o-x_lo_o)/(x_o-x_hi_o)^2-1/(x_o-x_hi_o))*(x_o-x_hi_o))/(x_o-x_lo_o);
diff_phi_x_o_y_o = 0;
diff_phi_x_o_theta_o = 0;

diff_phi_y_o_theta_1 = 0;
diff_phi_y_o_theta_2 = 0;
diff_phi_y_o_x_o = 0;
diff_phi_y_o_y_o = -(((y_o-y_lo_o)/(y_o-y_hi_o)^2-1/(y_o-y_hi_o))*(y_o-y_hi_o))/(y_o-y_lo_o);
diff_phi_y_o_theta_o = 0;

diff_phi_theta_o_theta_1 = 0;
diff_phi_theta_o_theta_2 = 0;
diff_phi_theta_o_x_o = 0;
diff_phi_theta_o_y_o = 0;
diff_phi_theta_o_theta_o = -(((theta_o-theta_lo_o)/(theta_o-theta_hi_o)^2-1/(theta_o-theta_hi_o))*(theta_o-theta_hi_o))/(theta_o-theta_lo_o);

chi_theta_1 = -((theta_1-theta_hi_1)*(thetadd_lo_1/(theta_1-theta_hi_1)-((theta_1-theta_lo_1)*thetadd_hi_1)/(theta_1-theta_hi_1)^2-(2*(thetad_1-thetad_hi_1)^2*(theta_1-theta_lo_1))/(theta_1-theta_hi_1)^3+(2*(thetad_1-thetad_hi_1)*(thetad_1-thetad_lo_1))/(theta_1-theta_hi_1)^2))/(theta_1-theta_lo_1)+(((thetad_1-thetad_lo_1)/(theta_1-theta_hi_1)-((thetad_1-thetad_hi_1)*(theta_1-theta_lo_1))/(theta_1-theta_hi_1)^2)*(thetad_1-thetad_hi_1))/(theta_1-theta_lo_1)-(((thetad_1-thetad_lo_1)/(theta_1-theta_hi_1)-((thetad_1-thetad_hi_1)*(theta_1-theta_lo_1))/(theta_1-theta_hi_1)^2)*(thetad_1-thetad_lo_1)*(theta_1-theta_hi_1))/(theta_1-theta_lo_1)^2;
chi_theta_2 = -((theta_2-theta_hi_2)*(thetadd_lo_2/(theta_2-theta_hi_2)-((theta_2-theta_lo_2)*thetadd_hi_2)/(theta_2-theta_hi_2)^2-(2*(thetad_2-thetad_hi_2)^2*(theta_2-theta_lo_2))/(theta_2-theta_hi_2)^3+(2*(thetad_2-thetad_hi_2)*(thetad_2-thetad_lo_2))/(theta_2-theta_hi_2)^2))/(theta_2-theta_lo_2)+(((thetad_2-thetad_lo_2)/(theta_2-theta_hi_2)-((thetad_2-thetad_hi_2)*(theta_2-theta_lo_2))/(theta_2-theta_hi_2)^2)*(thetad_2-thetad_hi_2))/(theta_2-theta_lo_2)-(((thetad_2-thetad_lo_2)/(theta_2-theta_hi_2)-((thetad_2-thetad_hi_2)*(theta_2-theta_lo_2))/(theta_2-theta_hi_2)^2)*(thetad_2-thetad_lo_2)*(theta_2-theta_hi_2))/(theta_2-theta_lo_2)^2;
chi_x_o = -((x_o-x_hi_o)*(xdd_lo_o/(x_o-x_hi_o)-((x_o-x_lo_o)*xdd_hi_o)/(x_o-x_hi_o)^2-(2*(xd_o-xd_hi_o)^2*(x_o-x_lo_o))/(x_o-x_hi_o)^3+(2*(xd_o-xd_hi_o)*(xd_o-xd_lo_o))/(x_o-x_hi_o)^2))/(x_o-x_lo_o)+(((xd_o-xd_lo_o)/(x_o-x_hi_o)-((xd_o-xd_hi_o)*(x_o-x_lo_o))/(x_o-x_hi_o)^2)*(xd_o-xd_hi_o))/(x_o-x_lo_o)-(((xd_o-xd_lo_o)/(x_o-x_hi_o)-((xd_o-xd_hi_o)*(x_o-x_lo_o))/(x_o-x_hi_o)^2)*(xd_o-xd_lo_o)*(x_o-x_hi_o))/(x_o-x_lo_o)^2;
chi_y_o = -((y_o-y_hi_o)*(ydd_lo_o/(y_o-y_hi_o)-((y_o-y_lo_o)*ydd_hi_o)/(y_o-y_hi_o)^2-(2*(yd_o-yd_hi_o)^2*(y_o-y_lo_o))/(y_o-y_hi_o)^3+(2*(yd_o-yd_hi_o)*(yd_o-yd_lo_o))/(y_o-y_hi_o)^2))/(y_o-y_lo_o)+(((yd_o-yd_lo_o)/(y_o-y_hi_o)-((yd_o-yd_hi_o)*(y_o-y_lo_o))/(y_o-y_hi_o)^2)*(yd_o-yd_hi_o))/(y_o-y_lo_o)-(((yd_o-yd_lo_o)/(y_o-y_hi_o)-((yd_o-yd_hi_o)*(y_o-y_lo_o))/(y_o-y_hi_o)^2)*(yd_o-yd_lo_o)*(y_o-y_hi_o))/(y_o-y_lo_o)^2;
chi_theta_o = -((theta_o-theta_hi_o)*(thetadd_lo_o/(theta_o-theta_hi_o)-((theta_o-theta_lo_o)*thetadd_hi_o)/(theta_o-theta_hi_o)^2-(2*(thetad_o-thetad_hi_o)^2*(theta_o-theta_lo_o))/(theta_o-theta_hi_o)^3+(2*(thetad_o-thetad_hi_o)*(thetad_o-thetad_lo_o))/(theta_o-theta_hi_o)^2))/(theta_o-theta_lo_o)+(((thetad_o-thetad_lo_o)/(theta_o-theta_hi_o)-((thetad_o-thetad_hi_o)*(theta_o-theta_lo_o))/(theta_o-theta_hi_o)^2)*(thetad_o-thetad_hi_o))/(theta_o-theta_lo_o)-(((thetad_o-thetad_lo_o)/(theta_o-theta_hi_o)-((thetad_o-thetad_hi_o)*(theta_o-theta_lo_o))/(theta_o-theta_hi_o)^2)*(thetad_o-thetad_lo_o)*(theta_o-theta_hi_o))/(theta_o-theta_lo_o)^2;


P = [diff_phi_theta_1_theta_1,diff_phi_theta_1_theta_2,diff_phi_theta_1_x_o,diff_phi_theta_1_y_o,diff_phi_theta_1_theta_o;
    diff_phi_theta_2_theta_1,diff_phi_theta_2_theta_2,diff_phi_theta_2_x_o,diff_phi_theta_2_y_o,diff_phi_theta_2_theta_o;
    diff_phi_x_o_theta_1,diff_phi_x_o_theta_2,diff_phi_x_o_x_o,diff_phi_x_o_y_o,diff_phi_x_o_theta_o;
    diff_phi_y_o_theta_1,diff_phi_y_o_theta_2,diff_phi_y_o_x_o,diff_phi_y_o_y_o,diff_phi_y_o_theta_o;
    diff_phi_theta_o_theta_1,diff_phi_theta_o_theta_2,diff_phi_theta_o_x_o,diff_phi_theta_o_y_o,diff_phi_theta_o_theta_o;];

chi = [chi_theta_1;chi_theta_2;chi_x_o;chi_y_o;chi_theta_o];

M_hat = M/P;

Q_hat = M/P*chi+QQ;

A = eye(5,5);
c = -gamma*[zeta1-zeta_ref_this1;
    zeta2-zeta_ref_this2;
    zeta3-zeta_ref_this3;
    zeta4-zeta_ref_this4;
    zeta5-zeta_ref_this5]+...
    [zetad_ref_this1;
    zetad_ref_this2;
    zetad_ref_this3;
    zetad_ref_this4;
    zetad_ref_this5];
b = -gamma*[zetad1-zetad_ref_this1;
    zetad2-zetad_ref_this2;
    zetad3-zetad_ref_this3;
    zetad4-zetad_ref_this4;
    zetad5-zetad_ref_this5]+...
    [zetadd_ref_this1;
    zetadd_ref_this2;
    zetadd_ref_this3;
    zetadd_ref_this4;
    zetadd_ref_this5];
zetad = [zetad1;zetad2;zetad3;zetad4;zetad5];

p1 = M_hat*(b-A/M_hat*Q_hat);
p2 = -kappa*M_hat*A.'/(A*A.')*(A*zetad-c);

PI = norm(zetad)+1;
% PI = abs(zetad1)+abs(zetad2)+abs(zetad3)+abs(zetad4)+abs(zetad5)+1;
beta = A*zetad-c;
alphad = k1*PI*norm(beta)-k2*alpha;
mu = beta*alpha*PI;
if(norm(mu)<epsilon)
    gamma = 1/epsilon;
else
    gamma = 1/norm(mu);
end
p4 = -M*A.'/(A*A.')*gamma*mu*alpha*PI;

UU = p1+p2+p4;
% UU = p1+p2;


UU1 = UU(1);
UU2 = UU(2);
UU3 = UU(3);
UU4 = UU(4);
UU5 = UU(5);

== matlab function CTS_inequality_2021b/Data sender ==
  data: t_ref_seq output; bound_seq output; bound_d_seq output; bound_dd_seq output; zeta_ref_seq output; zetad_ref_seq output; zetadd_ref_seq output
function [t_ref_seq,bound_seq,bound_d_seq,bound_dd_seq,zeta_ref_seq,zetad_ref_seq,zetadd_ref_seq] = fcn
coder.extrinsic('evalin');

L = 300;
t_ref_seq = zeros(1,L);
bound_seq = zeros(10,L);
bound_d_seq = zeros(10,L);
bound_dd_seq = zeros(10,L);
zeta_ref_seq = zeros(5,L);
zetad_ref_seq = zeros(5,L);
zetadd_ref_seq = zeros(5,L);

t_ref_seq = evalin('base','t_ref_seq');
bound_seq = evalin('base','bound_seq');
bound_d_seq = evalin('base','bound_d_seq');
bound_dd_seq = evalin('base','bound_dd_seq');
zeta_ref_seq = evalin('base','zeta_ref_seq');
zetad_ref_seq = evalin('base','zetad_ref_seq');
zetadd_ref_seq = evalin('base','zetadd_ref_seq');

== matlab function CTS_inequality_2021b/Force distribute ==
  data: xd_o input; yd_o input; theta_1 input; thetad_1 input; theta_2 input; thetad_2 input; theta_o input; thetad_o input; UU1 input; deltaf_1 output; deltam_1 output; UU2 input; UU3 input; UU4 input; UU5 input; deltar_1 output; Fxfl_1 output; Fxfr_1 output; Fxml_1 output; Fxmr_1 output; Fxrl_1 output; Fxrr_1 output; deltaf_2 output; deltam_2 output; deltar_2 output; Fxfl_2 output; Fxfr_2 output; Fxml_2 output; Fxmr_2 output; Fxrl_2 output; Fxrr_2 output; wx_1 input; wz_1 input; wx_2 input; wz_2 input; Fx_1 output; MZ_1 output; Fx_2 output; MZ_2 output
function [deltaf_1,deltam_1,deltar_1,Fxfl_1,Fxfr_1,Fxml_1,Fxmr_1,Fxrl_1,Fxrr_1,deltaf_2,deltam_2,deltar_2,Fxfl_2,Fxfr_2,Fxml_2,Fxmr_2,Fxrl_2,Fxrr_2,Fx_1,MZ_1,Fx_2,MZ_2] = fcn(xd_o,yd_o,theta_1,thetad_1,theta_2,thetad_2,theta_o,thetad_o,UU1,UU2,UU3,UU4,UU5,wx_1,wz_1,wx_2,wz_2)

a_1 = 1.11;
b_1 = 0.12;
c_1 = 1.23;
d_1 = 0.5;
r_1 = 5;
phip_1 = 0;
Cf_1 = -89752;
Cm_1 = -82100;
Cr_1 = -89752;

a_2 = 1.11;
b_2 = 0.12;
c_2 = 1.23;
d_2 = 0.5;
r_2 = 5;
phip_2 = pi;
Cf_2 = -86752;
Cm_2 = -83222;
Cr_2 = -86752;

T_1 = 1.5;
T_2 = 1.5;

xd_1 = xd_o-r_1*thetad_o*sin(theta_o+phip_1)+d_1*thetad_1*sin(theta_1);
yd_1 = yd_o+r_1*thetad_o*cos(theta_o+phip_1)-d_1*thetad_1*cos(theta_1);
xd_2 = xd_o-r_2*thetad_o*sin(theta_o+phip_2)+d_2*thetad_2*sin(theta_2);
yd_2 = yd_o+r_2*thetad_o*cos(theta_o+phip_2)-d_2*thetad_2*cos(theta_2);

u_1 = xd_1*cos(theta_1)+yd_1*sin(theta_1);
v_1 = -xd_1*sin(theta_1)+yd_1*cos(theta_1);
u_2 = xd_2*cos(theta_2)+yd_2*sin(theta_2);
v_2 = -xd_2*sin(theta_2)+yd_2*cos(theta_2);

C1_1 = -(2*Cf_1*(-sin(theta_1)+(v_1+a_1*thetad_1)/u_1*cos(theta_1))+2*Cm_1*(-sin(theta_1)+(v_1-b_1*thetad_1)/u_1*cos(theta_1))*(c_1-b_1)/(a_1+c_1));
C2_1 = -(2*Cr_1*(-sin(theta_1)+(v_1-c_1*thetad_1)/u_1*cos(theta_1))+2*Cm_1*(-sin(theta_1)+(v_1-b_1*thetad_1)/u_1*cos(theta_1))*(a_1+b_1)/(a_1+c_1));
C3_1 = 2*Cf_1*(-cos(theta_1)-(v_1+a_1*thetad_1)/u_1*sin(theta_1))+2*Cm_1*(-cos(theta_1)-(v_1-b_1*thetad_1)/u_1*sin(theta_1))*(c_1-b_1)/(a_1+c_1);
C4_1 = 2*Cr_1*(-cos(theta_1)-(v_1-c_1*thetad_1)/u_1*sin(theta_1))+2*Cm_1*(-cos(theta_1)-(v_1-b_1*thetad_1)/u_1*sin(theta_1))*(a_1+b_1)/(a_1+c_1);
C5_1 = -(2*Cf_1*a_1-2*Cm_1*b_1*(c_1-b_1)/(a_1+c_1));
C6_1 = 2*Cr_1*c_1+2*Cm_1*b_1*(a_1+b_1)/(a_1+c_1);

C1_2 = -(2*Cf_2*(-sin(theta_2)+(v_2+a_2*thetad_2)/u_2*cos(theta_2))+2*Cm_2*(-sin(theta_2)+(v_2-b_2*thetad_2)/u_2*cos(theta_2))*(c_2-b_2)/(a_2+c_2));
C2_2 = -(2*Cr_2*(-sin(theta_2)+(v_2-c_2*thetad_2)/u_2*cos(theta_2))+2*Cm_2*(-sin(theta_2)+(v_2-b_2*thetad_2)/u_2*cos(theta_2))*(a_2+b_2)/(a_2+c_2));
C3_2 = 2*Cf_2*(-cos(theta_2)-(v_2+a_2*thetad_2)/u_2*sin(theta_2))+2*Cm_2*(-cos(theta_2)-(v_2-b_2*thetad_2)/u_2*sin(theta_2))*(c_2-b_2)/(a_2+c_2);
C4_2 = 2*Cr_2*(-cos(theta_2)-(v_2-c_2*thetad_2)/u_2*sin(theta_2))+2*Cm_2*(-cos(theta_2)-(v_2-b_2*thetad_2)/u_2*sin(theta_2))*(a_2+b_2)/(a_2+c_2);
C5_2 = -(2*Cf_2*a_2-2*Cm_2*b_2*(c_2-b_2)/(a_2+c_2));
C6_2 = 2*Cr_2*c_2+2*Cm_2*b_2*(a_2+b_2)/(a_2+c_2);

J = [d_1*sin(theta_1) -d_1*cos(theta_1) 1 0 0 0;
    0 0 0 d_2*sin(theta_2) -d_2*cos(theta_2) 1;
    1 0 0 1 0 0;
    0 1 0 0 1 0;
    -r_1*sin(theta_o+phip_1) r_1*cos(theta_o+phip_1) 0 -r_2*sin(theta_o+phip_2) r_2*cos(theta_o+phip_2) 0];

U_xishu = [C1_1 C2_1 cos(theta_1) 0 0 0 0 0;
    C3_1 C4_1 sin(theta_1) 0 0 0 0 0;
    C5_1 C6_1 0 1 0 0 0 0;
    0 0 0 0 C1_2 C2_2 cos(theta_2) 0;
    0 0 0 0 C3_2 C4_2 sin(theta_2) 0;
    0 0 0 0 C5_2 C6_2 0 1];

B = J*U_xishu;


UU = [UU1;UU2;UU3;UU4;UU5];

W = diag([1e3,1e3,wx_1,wz_1,1e3,1e3,wx_2,wz_2]);
% tau = W\(B_cond.'*((B_cond*(W\B_cond.'))\UU));
ftau = zeros(size(B,2),1);
options = optimoptions('quadprog','Algorithm','active-set');
tau = quadprog(W,ftau,[],[],B,UU,[],[],zeros(8,1),options);

deltaf_1 = tau(1);
deltar_1 = tau(2);
deltam_1 = ((a_1+b_1)*deltar_1+(c_1-b_1)*deltaf_1)/(a_1+c_1);
Fx_1 = tau(3);
MZ_1 = tau(4);
deltaf_2 = tau(5);
deltar_2 = tau(6);
deltam_2 = ((a_2+b_2)*deltar_2+(c_2-b_2)*deltaf_2)/(a_2+c_2);
Fx_2 = tau(7);
MZ_2 = tau(8);

Dis_simple_1 = [1,1,1,1,1,1;
    -T_1/2,T_1/2,-T_1/2,T_1/2,-T_1/2,T_1/2];

Dis_simple_2 = [1,1,1,1,1,1;
    -T_2/2,T_2/2,-T_2/2,T_2/2,-T_2/2,T_2/2];

f = [];
A = [];
b = [];
F_min = -inf;
F_max = inf;
lb = [F_min;F_min;F_min;F_min;F_min;F_min];
ub = [F_max;F_max;F_max;F_max;F_max;F_max];
x0 = zeros(6,1);
options = optimoptions('quadprog','Algorithm','active-set');

H_1 = eye(6);
Fw_simple_1 = quadprog(H_1,f,A,b,Dis_simple_1,[Fx_1;MZ_1],lb,ub,x0,options);
Fxfl_1 = Fw_simple_1(1);
Fxfr_1 = Fw_simple_1(2);
Fxml_1 = Fw_simple_1(3);
Fxmr_1 = Fw_simple_1(4);
Fxrl_1 = Fw_simple_1(5);
Fxrr_1 = Fw_simple_1(6);

H_2 = eye(6);
Fw_simple_2 = quadprog(H_2,f,A,b,Dis_simple_2,[Fx_2;MZ_2],lb,ub,x0,options);
Fxfl_2 = Fw_simple_2(1);
Fxfr_2 = Fw_simple_2(2);
Fxml_2 = Fw_simple_2(3);
Fxmr_2 = Fw_simple_2(4);
Fxrl_2 = Fw_simple_2(5);
Fxrr_2 = Fw_simple_2(6);

== matlab function CTS_inequality_2021b/MATLAB Function ==
  data: t input; w1 output; w2 output; w3 output; w4 output
function [w1,w2,w3,w4] = fcn(t)

w1 = 1;
w2 = 1e4;
w3 = 1;
w4 = 1;

== matlab function CTS_inequality_2021b/Fxfl_disturb_1 ==
  data: u input; y output; t input
function y = fcn(u,t)

y = u+0.1*u*cos(0.2*t);

== matlab function CTS_inequality_2021b/Fxrl_disturb_2 ==
  data: u input; y output; t input
function y = fcn(u,t)

y = u+0.08*u*sin(0.32*t);

== matlab function CTS_inequality_2021b/Cal velocity ==
  data: u_1 output; theta_1 input; theta_2 input; theta_o input; Xd_o input; Yd_o input; thetad_1 input; phid_1 input; thetad_2 input; phid_2 input; thetad_o input; phid_o input; v_1 output; u_2 output; v_2 output; u_o output; v_o output
function [u_1,v_1,u_2,v_2,u_o,v_o] = fcn(theta_1,theta_2,theta_o,Xd_o,Yd_o,thetad_1,phid_1,thetad_2,phid_2,thetad_o,phid_o)

d_1 = 0.5;
r_1 = 5;
phip_1 = 0;
hcr_1 = 1;

d_2 = 0.5;
r_2 = 5;
phip_2 = pi;
hcr_2 = 1;

hr = 0.2;


u_o = Xd_o*cos(theta_o)+Yd_o*sin(theta_o);
v_o = Yd_o*cos(theta_o)-Xd_o*sin(theta_o);

u_1 = u_o*cos(theta_1-theta_o)+v_o*sin(theta_1-theta_o)-hcr_1*phid_o*sin(theta_1-theta_o)+hr*phid_o*sin(theta_1-theta_o)-r_1*thetad_o*sin(phip_1-theta_1+theta_o);
v_1 = hcr_1*phid_1-d_1*thetad_1-hr*phid_1+v_o*cos(theta_1-theta_o)-u_o*sin(theta_1-theta_o)-hcr_1*phid_o*cos(theta_1-theta_o)+hr*phid_o*cos(theta_1-theta_o)+r_1*thetad_o*cos(phip_1-theta_1+theta_o);

u_2 = u_o*cos(theta_2-theta_o)+v_o*sin(theta_2-theta_o)-hcr_2*phid_o*sin(theta_2-theta_o)+hr*phid_o*sin(theta_2-theta_o)-r_2*thetad_o*sin(phip_2-theta_2+theta_o);
v_2 = hcr_2*phid_2-d_2*thetad_2-hr*phid_2+v_o*cos(theta_2-theta_o)-u_o*sin(theta_2-theta_o)-hcr_2*phid_o*cos(theta_2-theta_o)+hr*phid_o*cos(theta_2-theta_o)+r_2*thetad_o*cos(phip_2-theta_2+theta_o);

end
